simulink model "ysw2sim_sine"  (Simulink 8.3)
settings: Solver=ode45  SolverMode=SingleTasking  StartTime=0.0  StopTime=50  FixedStep=0.001  RelTol=1e-3
settings Model: Creator=ljk  LastModifiedBy=ii  ExtModeTrigMode=oneshot  ExtModeArmWhenConnect=off
settings DataIOCC: LimitDataPoints=off  SignalLoggingName=sigsOut
settings OptimizationCC: BooleanDataType=off  ExpressionDepthLimit=2147483647
settings DebuggingCC: SaveWithParameterizedLinksMsg=none  SignalResolutionControl=TryResolveAllWithWarning  SolverPrmCheckMsg=none  MultiTaskDSMMsg=warning  MultiTaskCondExecSysMsg=none  FcnCallInpInsideContextMsg=UseLocalSettings
settings HardwareCC: TargetUnknown=on
settings RTWCC: IncludeERTFirstTime=on

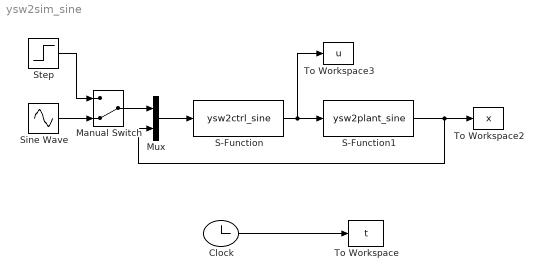
== system ysw2sim_sine ==
  Clock : Clock
  Manual Switch : ManualSwitch  CurrentSetting=0
  Mux : Mux  Inputs=2
  S-Function : S-Function  FunctionName=ysw2ctrl_sine  EnableBusSupport=off
  S-Function1 : S-Function  FunctionName=ysw2plant_sine  EnableBusSupport=off
  Sine Wave : Sin  SampleTime=0
  Step : Step  SampleTime=0
  To Workspace : ToWorkspace  VariableName=t  SampleTime=-1
  To Workspace2 : ToWorkspace  VariableName=x  SampleTime=-1
  To Workspace3 : ToWorkspace  VariableName=u  SampleTime=-1
  wires:
  Clock/1 -> To Workspace/1
  S-Function1/1 -> Mux/2, To Workspace2/1
  S-Function/1 -> To Workspace3/1, S-Function1/1
  Mux/1 -> S-Function/1
  Manual Switch/1 -> Mux/1
  Step/1 -> Manual Switch/1
  Sine Wave/1 -> Manual Switch/2
